simulink model "arcelik_a_senem_model"  (R2018b)
settings: Solver=FixedStepAuto  StartTime=0.0  StopTime=10  FixedStep=Tss  MaxStep=5e-5  RelTol=1e-3
undefined symbols (not defined in the file): Fs, polePairs, Tmax, Ts, Tss, Vdc, Wmax
libraries: simulink x1
settings Model: Creator=26046633  LastModifiedBy=26046633
settings SolverCC: ZeroCrossAlgorithm=Adaptive  AutoInsertRateTranBlk=on
settings DataIOCC: ReturnWorkspaceOutputs=on
settings DebuggingCC: IgnoredZcDiagnostic=none

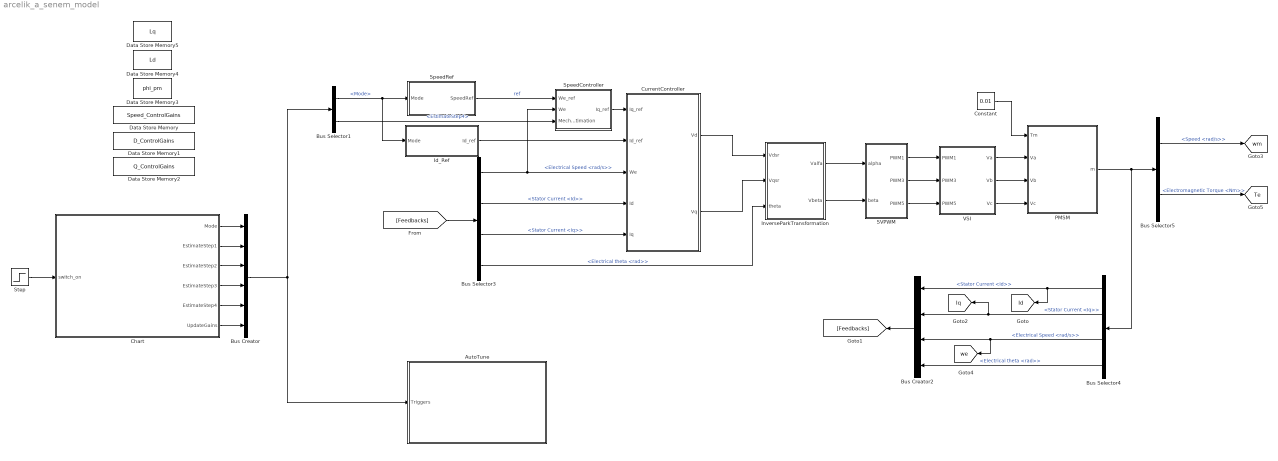
== system arcelik_a_senem_model ==
  AutoTune : Subsystem
  Bus Creator : BusCreator  Inputs=6
  Bus Creator2 : BusCreator  Inputs=4
  Bus Selector1 : BusSelector  OutputSignals=Mode,EstimateStep4
  Bus Selector3 : BusSelector  OutputSignals=Electrical Speed <rad/s>,Stator Current <Id>,Stator Current <Iq>,Electrical theta <rad>
  Bus Selector4 : BusSelector  OutputSignals=Stator Current <Id>,Stator Current <Iq>,Electrical Speed <rad/s>,Electrical theta <rad>
  Bus Selector5 : BusSelector  OutputSignals=Speed <rad/s>,Electromagnetic Torque <Nm>
  Chart : Stateflow chart  TreatAsAtomicUnit=on
  Constant : Constant  Value=0.01
  CurrentController : Subsystem
  Data Store Memory : DataStoreMemory  DataStoreName=Speed_ControlGains  InitialValue=[1 0]  ShowAdditionalParam=off
  Data Store Memory1 : DataStoreMemory  DataStoreName=D_ControlGains  InitialValue=[1 0]  ShowAdditionalParam=off
  Data Store Memory2 : DataStoreMemory  DataStoreName=Q_ControlGains  InitialValue=[1 0]  ShowAdditionalParam=off
  Data Store Memory3 : DataStoreMemory  DataStoreName=phi_pm  InitialValue=0.1  ShowAdditionalParam=off
  Data Store Memory4 : DataStoreMemory  DataStoreName=Ld  InitialValue=0.001  ShowAdditionalParam=off
  Data Store Memory5 : DataStoreMemory  DataStoreName=Lq  InitialValue=0.001  ShowAdditionalParam=off
  Id_Ref : Subsystem
  InverseParkTransformation : Subsystem
  PMSM : Subsystem  mask(Permanent Magnet Synchronous Motor :){Rs=7.1, Ld=30e-3, Lq=30e-3, flux=0.2, J=5.8e-4, B=2e-3, p=3}
      mask prompts: Rs "Stator Resistance - Rs [ohm] :"; Ld "Direct axis Inductance - Ld [H]"; Lq "Quadrature axis Inductance - Lq [H] :"; flux "Flux - [Wb]"; J "Rotor Inertia - J [kg-m^2]"; B "Friction Coefficient - B"; p "Number of Pole Pairs"
      mask Display: fprintf('PMSM')
  SVPWM : Subsystem
  SpeedController : Subsystem
  SpeedRef : Subsystem
  Step : Step  Time=3  Before=1  After=0  SampleTime=0
  VSI : Subsystem
  tag scope: Id=global, Iq=global, Te=global, we=global, wm=global
  wires:
  SVPWM/3(PWM5) -> VSI/3(PWM5)
  SVPWM/1(PWM1) -> VSI/1(PWM1)
  SVPWM/2(PWM3) -> VSI/2(PWM3)
  VSI/1(Va) -> PMSM/2(Va)
  VSI/2(Vb) -> PMSM/3(Vb)
  VSI/3(Vc) -> PMSM/4(Vc)
  SpeedController/1(Iq_ref) -> CurrentController/1(Iq_ref)
  SpeedRef/1(SpeedRef) -> SpeedController/1(We_ref)  "ref"
  Step/1 -> Chart/1(switch_on)
  Id_Ref/1(Id_ref) -> CurrentController/2(Id_ref)
  Chart/1(Mode) -> Bus Creator/1
  Chart/2(EstimateStep1) -> Bus Creator/2
  Chart/3(EstimateStep2) -> Bus Creator/3
  Chart/4(EstimateStep3) -> Bus Creator/4
  Bus Creator/1 -> AutoTune/1(Triggers), Bus Selector1/1
  Bus Selector1/1 -> Id_Ref/1(Mode), SpeedRef/1(Mode)  "<Mode>"
  [Feedbacks] -> Bus Selector3/1
  Bus Selector3/4 -> InverseParkTransformation/3(theta)  "<Electrical theta <rad>>"
  Bus Selector3/1 -> SpeedController/2(We), CurrentController/3(We)  "<Electrical Speed <rad/s>>"
  Bus Selector3/2 -> CurrentController/4(Id)  "<Stator Current <Id>>"
  Bus Selector3/3 -> CurrentController/5(Iq)  "<Stator Current <Iq>>"
  PMSM/1(m) -> Bus Selector4/1, Bus Selector5/1
  InverseParkTransformation/1(Valfa) -> SVPWM/1(alpha)
  InverseParkTransformation/2(Vbeta) -> SVPWM/2(beta)
  CurrentController/2(Vq) -> InverseParkTransformation/2(Vqsr)
  CurrentController/1(Vd) -> InverseParkTransformation/1(Vdsr)
  Bus Creator2/1 -> [Feedbacks]
  Constant/1 -> PMSM/1(Tm)
  Bus Selector4/1 -> Bus Creator2/1, [Id]  "<Stator Current <Id>>"
  Bus Selector4/4 -> Bus Creator2/4  "<Electrical theta <rad>>"
  Bus Selector4/3 -> Bus Creator2/3, [we]  "<Electrical Speed <rad/s>>"
  Bus Selector4/2 -> [Iq], Bus Creator2/2  "<Stator Current <Iq>>"
  Bus Selector5/2 -> [Te]  "<Electromagnetic Torque <Nm>>"
  Bus Selector1/2 -> SpeedController/3(MechanicalEstimation)  "<EstimateStep4>"
  Bus Selector5/1 -> [wm]  "<Speed <rad/s>>"
  Chart/5(EstimateStep4) -> Bus Creator/5
  Chart/6(UpdateGains) -> Bus Creator/6

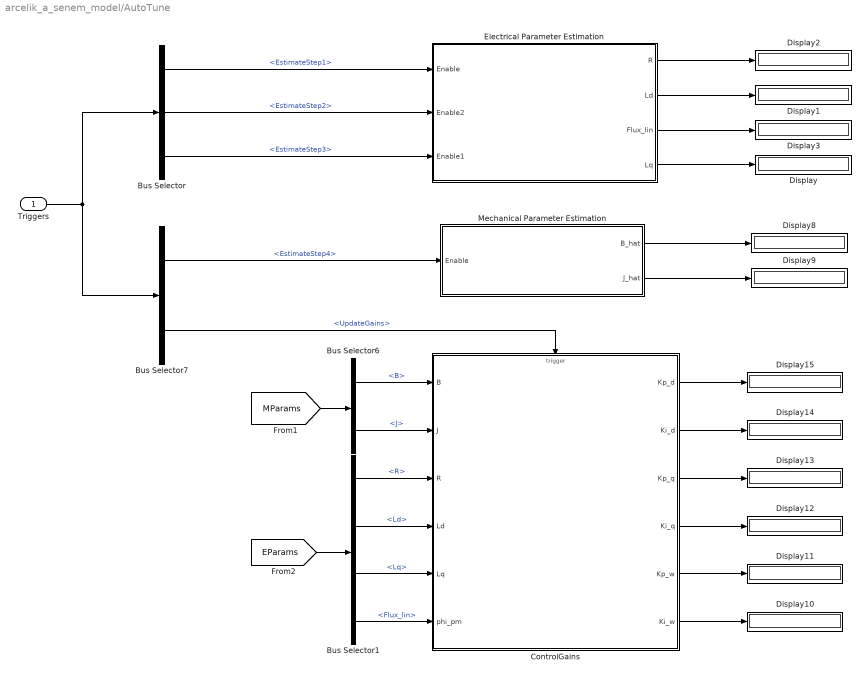
== system arcelik_a_senem_model/AutoTune ==
  Triggers : Inport
  Bus Selector : BusSelector  OutputSignals=EstimateStep1,EstimateStep2,EstimateStep3
  Bus Selector1 : BusSelector  OutputSignals=R,Ld,Lq,Flux_lin
  Bus Selector6 : BusSelector  OutputSignals=B,J
  Bus Selector7 : BusSelector  OutputSignals=EstimateStep4,UpdateGains
  ControlGains : Subsystem
  Display{,1..3,8..15} (12 alike) : Display
      Display1 settings: Decimation=4
  Electrical Parameter Estimation : Subsystem
  Mechanical Parameter Estimation : Subsystem
  wires:
  ControlGains/5(Kp_w) -> Display11/1
  Bus Selector/2 -> Electrical Parameter Estimation/2(Enable2)  "<EstimateStep2>"
  Electrical Parameter Estimation/2(Ld) -> Display1/1
  Mechanical Parameter Estimation/2(J_hat) -> Display9/1
  Electrical Parameter Estimation/1(R) -> Display2/1
  Bus Selector7/1 -> Mechanical Parameter Estimation/1(Enable)  "<EstimateStep4>"
  Bus Selector/3 -> Electrical Parameter Estimation/3(Enable1)  "<EstimateStep3>"
  Bus Selector/1 -> Electrical Parameter Estimation/1(Enable)  "<EstimateStep1>"
  Electrical Parameter Estimation/3(Flux_lin) -> Display3/1
  Electrical Parameter Estimation/4(Lq) -> Display/1
  Triggers/1 -> Bus Selector/1, Bus Selector7/1
  ControlGains/6(Ki_w) -> Display10/1
  [MParams] -> Bus Selector6/1
  Mechanical Parameter Estimation/1(B_hat) -> Display8/1
  Bus Selector7/2 -> ControlGains/Trigger  "<UpdateGains>"
  Bus Selector1/3 -> ControlGains/5(Lq)  "<Lq>"
  Bus Selector1/2 -> ControlGains/4(Ld)  "<Ld>"
  [EParams] -> Bus Selector1/1
  Bus Selector1/1 -> ControlGains/3(R)  "<R>"
  ControlGains/4(Ki_q) -> Display12/1
  ControlGains/3(Kp_q) -> Display13/1
  ControlGains/2(Ki_d) -> Display14/1
  ControlGains/1(Kp_d) -> Display15/1
  Bus Selector6/1 -> ControlGains/1(B)  "<B>"
  Bus Selector6/2 -> ControlGains/2(J)  "<J>"
  Bus Selector1/4 -> ControlGains/6(phi_pm)  "<Flux_lin>"

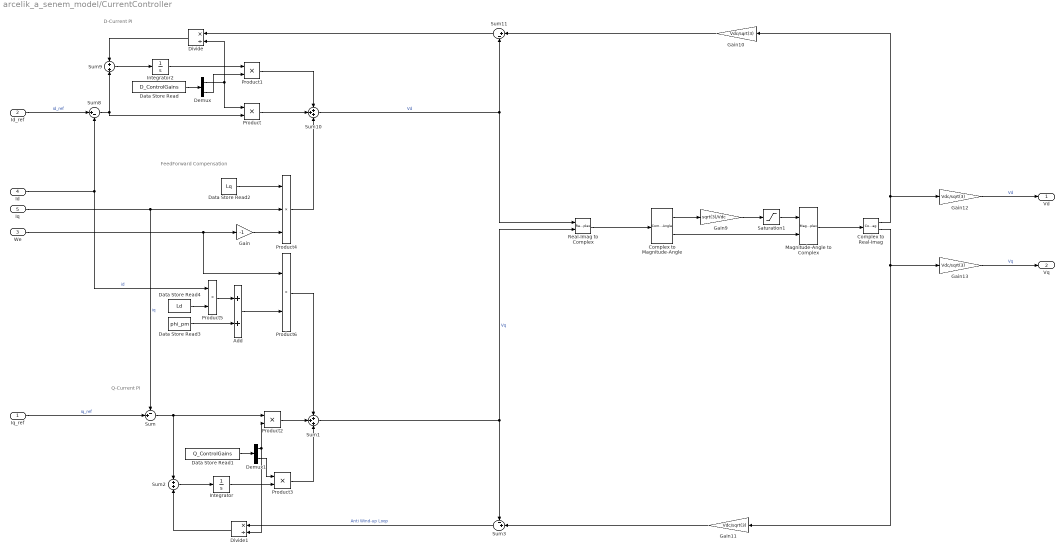
== system arcelik_a_senem_model/CurrentController ==
  note: FeedForward Compensation
  note: Q-Current PI
  note: D-Current PI
  Iq_ref : Inport
  Id_ref : Inport  Port=2
  We : Inport  Port=3
  Id : Inport  Port=4
  Iq : Inport  Port=5
  Add : Sum
  Complex to Magnitude-Angle : ComplexToMagnitudeAngle
  Complex to Real-Imag : ComplexToRealImag
  Data Store Read : DataStoreRead  DataStoreName=D_ControlGains
  Data Store Read1 : DataStoreRead  DataStoreName=Q_ControlGains
  Data Store Read2 : DataStoreRead  DataStoreName=Lq
  Data Store Read3 : DataStoreRead  DataStoreName=phi_pm
  Data Store Read4 : DataStoreRead  DataStoreName=Ld
  Demux : Demux  Outputs=2
  Demux1 : Demux  Outputs=2
  Divide : Product  Inputs=*/
  Divide1 : Product  Inputs=*/
  Gain : Gain  Gain=-1
  Gain{10..13} (4 alike) : Gain  Gain=Vdc/sqrt(3)
  Gain9 : Gain  Gain=sqrt(3)/Vdc
  Integrator : Integrator
  Integrator2 : Integrator
  Magnitude-Angle to Complex : MagnitudeAngleToComplex
  Product{,1..3,5..6} (6 alike) : Product
  Product4 : Product  Inputs=3
  Real-Imag to Complex : RealImagToComplex
  Saturation1 : Saturate  UpperLimit=sqrt(3)*2/3  LowerLimit=-sqrt(3)*2/3
  Sum : Sum  Inputs=-+|
  Sum1 : Sum  Inputs=+++
  Sum10 : Sum  Inputs=+++
  Sum11 : Sum  Inputs=|+-
  Sum2 : Sum
  Sum3 : Sum  Inputs=-+|
  Sum8 : Sum  Inputs=|+-
  Sum9 : Sum  Inputs=+|+
  Vd : Outport
  Vq : Outport  Port=2
  wires:
  Integrator2/1 -> Product1/1
  Sum/1 -> Sum2/1, Product2/1
  Product6/1 -> Sum1/1
  Integrator/1 -> Product3/2
  Sum2/1 -> Integrator/1
  Sum8/1 -> Product/2, Sum9/2
  Product4/1 -> Sum10/3
  Product3/1 -> Sum1/3
  Id/1 -> Sum8/2, Product5/1  "id"
  Divide/1 -> Sum9/1
  Iq/1 -> Sum/1, Product4/2  "iq"
  Product1/1 -> Sum10/1
  Product2/1 -> Sum1/2
  Divide1/1 -> Sum2/2
  Id_ref/1 -> Sum8/1  "id_ref"
  Sum9/1 -> Integrator2/1
  Product/1 -> Sum10/2
  We/1 -> Product6/1, Gain/1
  Complex to Magnitude-Angle/2 -> Magnitude-Angle to Complex/2
  Sum11/1 -> Divide/1
  Gain11/1 -> Sum3/2
  Real-Imag to Complex/1 -> Complex to Magnitude-Angle/1
  Gain10/1 -> Sum11/1
  Gain9/1 -> Saturation1/1
  Complex to Magnitude-Angle/1 -> Gain9/1
  Gain13/1 -> Vq/1  "Vq"
  Sum3/1 -> Divide1/1  "Anti Wind-up Loop"
  Complex to Real-Imag/2 -> Gain13/1, Gain11/1
  Sum1/1 -> Sum3/1, Real-Imag to Complex/2  "Vq"
  Complex to Real-Imag/1 -> Gain10/1, Gain12/1
  Magnitude-Angle to Complex/1 -> Complex to Real-Imag/1
  Sum10/1 -> Real-Imag to Complex/1, Sum11/2  "Vd"
  Saturation1/1 -> Magnitude-Angle to Complex/1
  Iq_ref/1 -> Sum/2  "iq_ref"
  Gain12/1 -> Vd/1  "Vd"
  Data Store Read/1 -> Demux/1
  Demux/1 -> Divide/2, Product/1
  Demux/2 -> Product1/2
  Data Store Read1/1 -> Demux1/1
  Demux1/1 -> Product2/2, Divide1/2
  Demux1/2 -> Product3/1
  Data Store Read2/1 -> Product4/1
  Gain/1 -> Product4/3
  Data Store Read4/1 -> Product5/2
  Product5/1 -> Add/1
  Data Store Read3/1 -> Add/2
  Add/1 -> Product6/2

== system arcelik_a_senem_model/Id_Ref ==
  Mode : Inport
  Constant1 : Constant  Value=0
  Multiport Switch1 : MultiPortSwitch  Inputs=4
  Sine Wave : Sin  Amplitude=0.1  Frequency=100*2*pi  SampleTime=0
  Sine Wave1 : Sin  Amplitude=0.1  Frequency=500*2*pi  SampleTime=0
  Sum : Sum
  Id_ref : Outport
  wires:
  Multiport Switch1/1 -> Id_ref/1
  Sum/1 -> Multiport Switch1/2
  Sine Wave/1 -> Sum/1
  Sine Wave1/1 -> Sum/2
  Mode/1 -> Multiport Switch1/1
  Constant1/1 -> Multiport Switch1/5, Multiport Switch1/4, Multiport Switch1/3

== system arcelik_a_senem_model/InverseParkTransformation ==
  Vdsr : Inport
  Vqsr : Inport  Port=2
  theta : Inport  Port=3
  ipark : MATLAB Function  TreatAsAtomicUnit=on  SystemSampleTime=Ts
  Valfa : Outport  VectorParamsAs1DForOutWhenUnconnected=off
  Vbeta : Outport  Port=2  VectorParamsAs1DForOutWhenUnconnected=off
  wires:
  theta/1 -> ipark/3(Angle)
  ipark/1(Alpha) -> Valfa/1
  ipark/2(Beta) -> Vbeta/1
  Vdsr/1 -> ipark/1(Ds)
  Vqsr/1 -> ipark/2(Qs)

== system arcelik_a_senem_model/PMSM ==
  Tm : Inport
  Va : Inport  Port=2
  Vb : Inport  Port=3
  Vc : Inport  Port=4
  Clark & Park Tranformations : Subsystem
  "Id, Iq Calculation" : Subsystem
  Mechanical Calculation : Subsystem
  Torque Calculation : Subsystem
  measurement : Subsystem
  m : Outport
  tag scope: Vd=global, Vq=global
  wires:
  Tm/1 -> Mechanical Calculation/2(Tm)
  Torque Calculation/1(Te) -> measurement/3(Te), Mechanical Calculation/1(Te)
  Mechanical Calculation/4(we) -> "Id, Iq Calculation"/3(we), measurement/7(we)
  Mechanical Calculation/3(theta) -> Clark & Park Tranformations/4(theta), measurement/6(theta_e)
  "Id, Iq Calculation"/1(Iq) -> measurement/2(Iq), Torque Calculation/1(Iq)
  Mechanical Calculation/1(wm) -> measurement/4(wm)
  Mechanical Calculation/2(theta m) -> measurement/5(theta_m)
  measurement/1(m) -> m/1
  Clark & Park Tranformations/1(Vq) -> [Vq], "Id, Iq Calculation"/1(Vq)
  Clark & Park Tranformations/2(Vd) -> [Vd], "Id, Iq Calculation"/2(Vd)
  Va/1 -> Clark & Park Tranformations/1(Va)
  Vc/1 -> Clark & Park Tranformations/3(Vc)
  Vb/1 -> Clark & Park Tranformations/2(Vb)
  "Id, Iq Calculation"/2(Id) -> measurement/1(Id), Torque Calculation/2(Id)

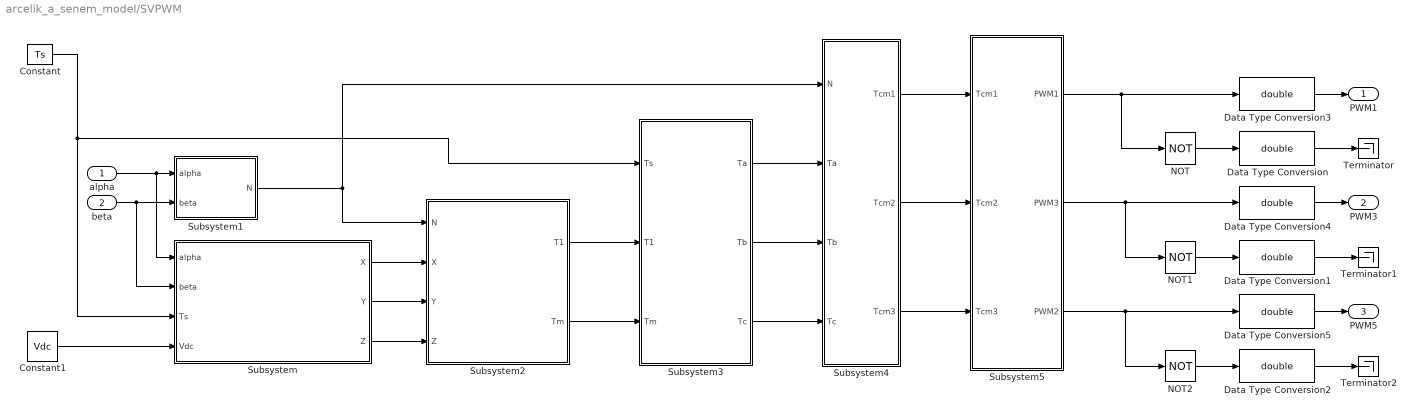
== system arcelik_a_senem_model/SVPWM ==
  alpha : Inport
  beta : Inport  Port=2
  Constant : Constant  Value=Ts
  Constant1 : Constant  Value=Vdc
  Data Type Conversion{,1..5} (6 alike) : DataTypeConversion  OutDataTypeStr=double
  NOT : Logic  Operator=NOT  AllPortsSameDT=off  OutDataTypeStr=boolean
  NOT1 : Logic  Operator=NOT  AllPortsSameDT=off  OutDataTypeStr=boolean
  NOT2 : Logic  Operator=NOT  AllPortsSameDT=off  OutDataTypeStr=boolean
  Subsystem : Subsystem
  Subsystem1 : Subsystem
  Subsystem2 : Subsystem
  Subsystem3 : Subsystem
  Subsystem4 : Subsystem
  Subsystem5 : Subsystem
  Terminator : Terminator
  Terminator1 : Terminator
  Terminator2 : Terminator
  PWM1 : Outport
  PWM3 : Outport  Port=2
  PWM5 : Outport  Port=3
  wires:
  Subsystem5/3(PWM2) -> Data Type Conversion5/1, NOT2/1
  NOT2/1 -> Data Type Conversion2/1
  NOT1/1 -> Data Type Conversion1/1
  NOT/1 -> Data Type Conversion/1
  Subsystem3/3(Tc) -> Subsystem4/4(Tc)
  Subsystem3/1(Ta) -> Subsystem4/2(Ta)
  Subsystem5/2(PWM3) -> Data Type Conversion4/1, NOT1/1
  Subsystem5/1(PWM1) -> Data Type Conversion3/1, NOT/1
  Subsystem4/3(Tcm3) -> Subsystem5/3(Tcm3)
  Subsystem4/2(Tcm2) -> Subsystem5/2(Tcm2)
  Subsystem4/1(Tcm1) -> Subsystem5/1(Tcm1)
  Subsystem3/2(Tb) -> Subsystem4/3(Tb)
  Constant/1 -> Subsystem3/1(Ts), Subsystem/3(Ts)
  Constant1/1 -> Subsystem/4(Vdc)
  beta/1 -> Subsystem1/2(beta), Subsystem/2(beta)
  Subsystem1/1(N) -> Subsystem4/1(N), Subsystem2/1(N)
  alpha/1 -> Subsystem1/1(alpha), Subsystem/1(alpha)
  Subsystem/2(Y) -> Subsystem2/3(Y)
  Subsystem/1(X) -> Subsystem2/2(X)
  Subsystem2/2(Tm) -> Subsystem3/3(Tm)
  Subsystem2/1(T1) -> Subsystem3/2(T1)
  Subsystem/3(Z) -> Subsystem2/4(Z)
  Data Type Conversion3/1 -> PWM1/1
  Data Type Conversion4/1 -> PWM3/1
  Data Type Conversion5/1 -> PWM5/1
  Data Type Conversion/1 -> Terminator/1
  Data Type Conversion1/1 -> Terminator1/1
  Data Type Conversion2/1 -> Terminator2/1

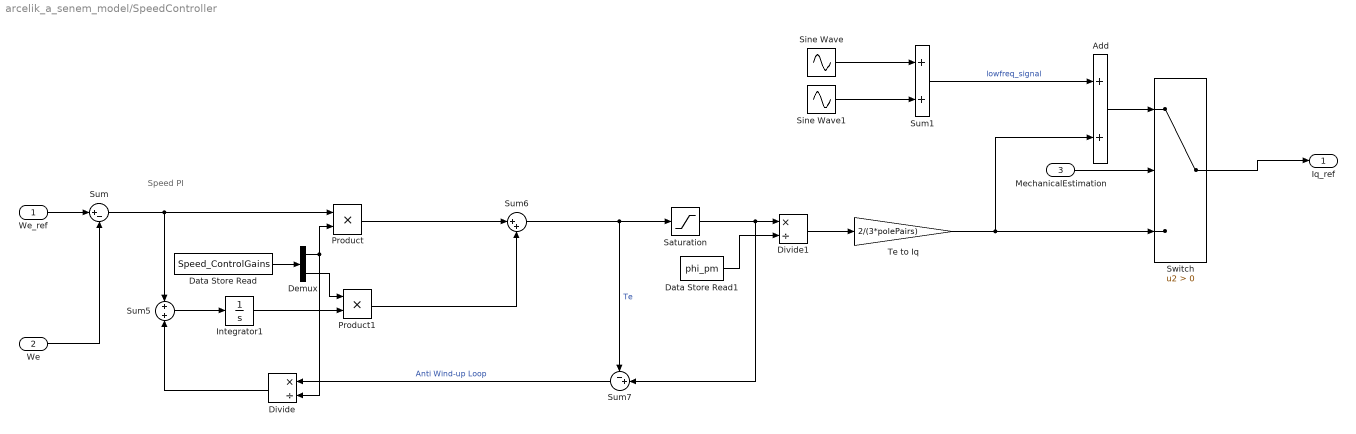
== system arcelik_a_senem_model/SpeedController ==
  note: Speed PI
  We_ref : Inport
  We : Inport  Port=2
  MechanicalEstimation : Inport  Port=3
  Add : Sum
  Data Store Read : DataStoreRead  DataStoreName=Speed_ControlGains
  Data Store Read1 : DataStoreRead  DataStoreName=phi_pm
  Demux : Demux  Outputs=2
  Divide : Product  Inputs=*/
  Divide1 : Product  Inputs=*/
  Integrator1 : Integrator
  Product : Product
  Product1 : Product
  Saturation : Saturate  UpperLimit=Tmax  LowerLimit=-Tmax
  Sine Wave : Sin  Amplitude=0.1  Frequency=0.1*2*pi  SampleTime=0
  Sine Wave1 : Sin  Amplitude=0.1  Frequency=0.25*2*pi  SampleTime=0
  Sum : Sum  Inputs=|+-
  Sum1 : Sum
  Sum5 : Sum
  Sum6 : Sum  Inputs=|++
  Sum7 : Sum  Inputs=-+|
  Switch : Switch  Criteria=u2 > Threshold
  Te to Iq : Gain  Gain=2/(3*polePairs)
  Iq_ref : Outport
  wires:
  Product1/1 -> Sum6/2
  Sum5/1 -> Integrator1/1
  Saturation/1 -> Sum7/2, Divide1/1
  Integrator1/1 -> Product1/2
  Sum6/1 -> Saturation/1, Sum7/1  "Te"
  Sum7/1 -> Divide/1  "Anti Wind-up Loop"
  Product/1 -> Sum6/1
  Divide/1 -> Sum5/2
  Sum/1 -> Sum5/1, Product/1
  We_ref/1 -> Sum/1
  We/1 -> Sum/2
  Te to Iq/1 -> Add/2, Switch/3
  Switch/1 -> Iq_ref/1
  Sine Wave1/1 -> Sum1/2
  Sine Wave/1 -> Sum1/1
  MechanicalEstimation/1 -> Switch/2
  Add/1 -> Switch/1
  Sum1/1 -> Add/1  "lowfreq_signal"
  Data Store Read/1 -> Demux/1
  Demux/2 -> Product1/1
  Demux/1 -> Product/2, Divide/2
  Divide1/1 -> Te to Iq/1
  Data Store Read1/1 -> Divide1/2

== system arcelik_a_senem_model/SpeedRef ==
  Mode : Inport
  Constant : Constant  Value=100
  Constant1 : Constant  Value=2500
  Constant2 : Constant  Value=Wmax
  Constant3 : Constant  Value=0
  Gain : Gain  Gain=Wmax
  Gain1 : Gain  Gain=pi/(30*Wmax)
  Gain2 : Gain  Gain=pi/(30*Wmax)
  Gain3 : Gain  Gain=pi/(30*Wmax)
  Multiport Switch : MultiPortSwitch  Inputs=4
  RC_MACRO1 : MATLAB Function  TreatAsAtomicUnit=on  SystemSampleTime=Ts
  Step : Step  Time=5.5  After=1000  SampleTime=0
  SpeedRef : Outport
  wires:
  Constant/1 -> Gain1/1  "rpm"
  Mode/1 -> Multiport Switch/1
  Constant3/1 -> Multiport Switch/2
  Step/1 -> Gain3/1
  Constant1/1 -> Gain2/1  "rpm"
  RC_MACRO1/1(SetpointValue) -> Gain/1
  Multiport Switch/1 -> RC_MACRO1/1(inp)  "rad/s"
  Constant2/1 -> RC_MACRO1/2(MaxSpeed)
  Gain/1 -> SpeedRef/1
  Gain1/1 -> Multiport Switch/3  "rad/s"
  Gain2/1 -> Multiport Switch/4  "rad/s"
  Gain3/1 -> Multiport Switch/5  "rad/s"

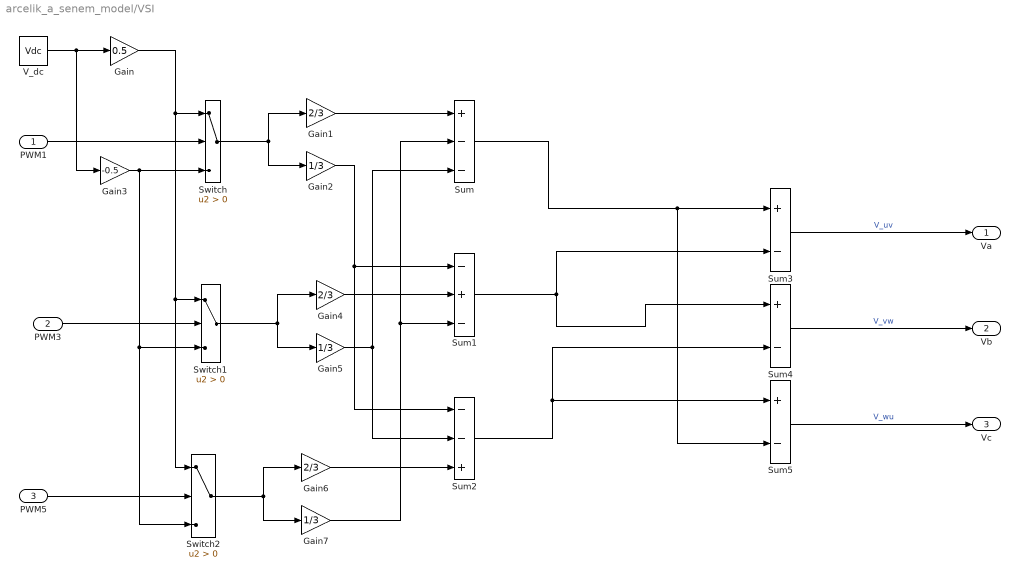
== system arcelik_a_senem_model/VSI ==
  PWM1 : Inport
  PWM3 : Inport  Port=2
  PWM5 : Inport  Port=3
  Gain : Gain  Gain=0.5
  Gain1 : Gain  Gain=2/3
  Gain2 : Gain  Gain=1/3
  Gain3 : Gain  Gain=-0.5
  Gain4 : Gain  Gain=2/3
  Gain5 : Gain  Gain=1/3
  Gain6 : Gain  Gain=2/3
  Gain7 : Gain  Gain=1/3
  Sum : Sum  Inputs=+--
  Sum1 : Sum  Inputs=-+-
  Sum2 : Sum  Inputs=--+
  Sum3 : Sum  Inputs=+-
  Sum4 : Sum  Inputs=+-
  Sum5 : Sum  Inputs=+-
  Switch : Switch  Criteria=u2 > Threshold
  Switch1 : Switch  Criteria=u2 > Threshold
  Switch2 : Switch  Criteria=u2 > Threshold
  V_dc : Constant  Value=Vdc
  Va : Outport
  Vb : Outport  Port=2
  Vc : Outport  Port=3
  wires:
  V_dc/1 -> Gain3/1, Gain/1
  PWM1/1 -> Switch/2
  Switch/1 -> Gain2/1, Gain1/1
  Gain1/1 -> Sum/1
  Sum/1 -> Sum5/2, Sum3/1
  PWM3/1 -> Switch1/2
  Sum1/1 -> Sum3/2, Sum4/1
  Switch1/1 -> Gain4/1, Gain5/1
  Gain4/1 -> Sum1/2
  Switch2/1 -> Gain7/1, Gain6/1
  Sum2/1 -> Sum4/2, Sum5/1
  Gain3/1 -> Switch2/3, Switch1/3, Switch/3
  PWM5/1 -> Switch2/2
  Gain/1 -> Switch2/1, Switch1/1, Switch/1
  Gain6/1 -> Sum2/3
  Gain7/1 -> Sum1/3, Sum/2
  Gain5/1 -> Sum/3, Sum2/2
  Gain2/1 -> Sum2/1, Sum1/1
  Sum3/1 -> Va/1  "V_uv"
  Sum4/1 -> Vb/1  "V_vw"
  Sum5/1 -> Vc/1  "V_wu"

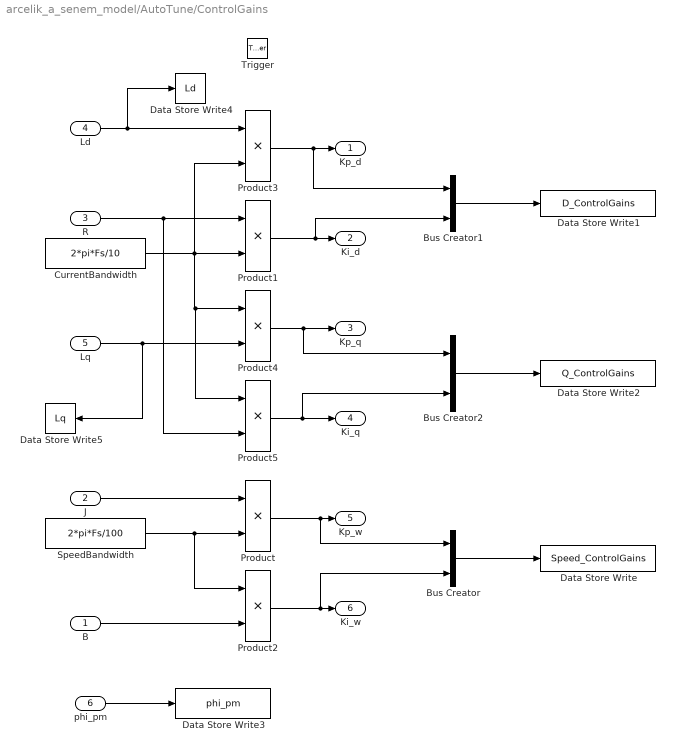
== system arcelik_a_senem_model/AutoTune/ControlGains ==
  B : Inport
  J : Inport  Port=2
  R : Inport  Port=3
  Ld : Inport  Port=4
  Lq : Inport  Port=5
  phi_pm : Inport  Port=6
  Trigger : TriggerPort  VariantControl=Variant  PortDimensions=1
  Bus Creator : BusCreator  Inputs=2
  Bus Creator1 : BusCreator  Inputs=2
  Bus Creator2 : BusCreator  Inputs=2
  CurrentBandwidth : Constant  Value=2*pi*Fs/10
  Data Store Write : DataStoreWrite  DataStoreName=Speed_ControlGains
  Data Store Write1 : DataStoreWrite  DataStoreName=D_ControlGains
  Data Store Write2 : DataStoreWrite  DataStoreName=Q_ControlGains
  Data Store Write3 : DataStoreWrite  DataStoreName=phi_pm
  Data Store Write4 : DataStoreWrite  DataStoreName=Ld
  Data Store Write5 : DataStoreWrite  DataStoreName=Lq
  Product{,1..5} (6 alike) : Product
  SpeedBandwidth : Constant  Value=2*pi*Fs/100
  Kp_d : Outport
  Ki_d : Outport  Port=2
  Kp_q : Outport  Port=3
  Ki_q : Outport  Port=4
  Kp_w : Outport  Port=5
  Ki_w : Outport  Port=6
  wires:
  B/1 -> Product2/2
  SpeedBandwidth/1 -> Product/2, Product2/1
  J/1 -> Product/1
  Bus Creator/1 -> Data Store Write/1
  Product2/1 -> Bus Creator/2, Ki_w/1
  Bus Creator1/1 -> Data Store Write1/1
  Bus Creator2/1 -> Data Store Write2/1
  Lq/1 -> Data Store Write5/1, Product4/2
  Product5/1 -> Bus Creator2/2, Ki_q/1
  Ld/1 -> Data Store Write4/1, Product3/1
  CurrentBandwidth/1 -> Product5/1, Product4/1, Product3/2, Product1/2
  Product1/1 -> Bus Creator1/2, Ki_d/1
  R/1 -> Product5/2, Product1/1
  Product3/1 -> Bus Creator1/1, Kp_d/1
  Product4/1 -> Bus Creator2/1, Kp_q/1
  Product/1 -> Bus Creator/1, Kp_w/1
  phi_pm/1 -> Data Store Write3/1

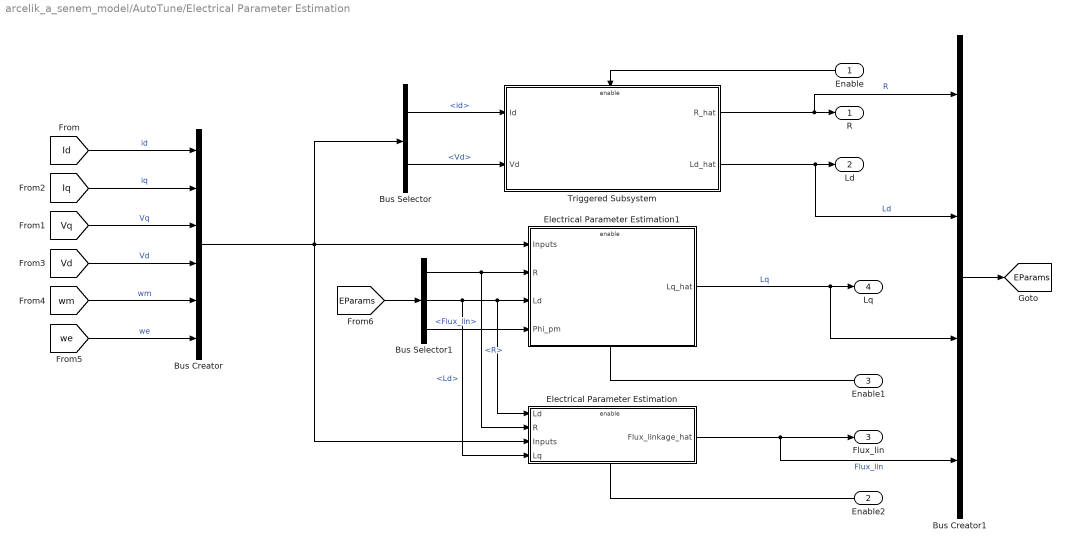
== system arcelik_a_senem_model/AutoTune/Electrical Parameter Estimation ==
  Enable : Inport
  Enable2 : Inport  Port=2
  Enable1 : Inport  Port=3
  Bus Creator : BusCreator  Inputs=6
  Bus Creator1 : BusCreator  Inputs=4
  Bus Selector : BusSelector  OutputSignals=id,Vd
  Bus Selector1 : BusSelector  OutputSignals=R,Ld,Flux_lin
  Electrical Parameter Estimation : Subsystem
  Electrical Parameter Estimation1 : Subsystem
  Triggered Subsystem : Subsystem  TreatAsAtomicUnit=on
  R : Outport
  Ld : Outport  Port=2
  Flux_lin : Outport  Port=3
  Lq : Outport  Port=4
  tag scope: EParams=global
  wires:
  [Vq] -> Bus Creator/3  "Vq"
  Bus Creator/1 -> Electrical Parameter Estimation/3(Inputs), Electrical Parameter Estimation1/1(Inputs), Bus Selector/1
  [we] -> Bus Creator/6  "we"
  [Id] -> Bus Creator/1  "id"
  [wm] -> Bus Creator/5  "wm"
  Bus Selector/1 -> Triggered Subsystem/1(Id)  "<id>"
  [Iq] -> Bus Creator/2  "iq"
  Bus Selector/2 -> Triggered Subsystem/2(Vd)  "<Vd>"
  Enable1/1 -> Electrical Parameter Estimation1/Enable
  [Vd] -> Bus Creator/4  "Vd"
  Electrical Parameter Estimation/1(Flux_linkage_hat) -> Flux_lin/1, Bus Creator1/4  "Flux_lin"
  Enable2/1 -> Electrical Parameter Estimation/Enable
  Electrical Parameter Estimation1/1(Lq_hat) -> Bus Creator1/3, Lq/1  "Lq"
  Triggered Subsystem/1(R_hat) -> Bus Creator1/1, R/1  "R"
  Triggered Subsystem/2(Ld_hat) -> Bus Creator1/2, Ld/1  "Ld"
  Bus Creator1/1 -> [EParams]
  [EParams] -> Bus Selector1/1
  Bus Selector1/1 -> Electrical Parameter Estimation/2(R), Electrical Parameter Estimation1/2(R)  "<R>"
  Bus Selector1/2 -> Electrical Parameter Estimation/4(Lq), Electrical Parameter Estimation/1(Ld), Electrical Parameter Estimation1/3(Ld)  "<Ld>"
  Bus Selector1/3 -> Electrical Parameter Estimation1/4(Phi_pm)  "<Flux_lin>"
  Enable/1 -> Triggered Subsystem/Enable

== system arcelik_a_senem_model/AutoTune/Mechanical Parameter Estimation ==
  Enable : Inport
  Bus Creator : BusCreator  Inputs=2
  Mechanical Parameter Estimation : Subsystem
  B_hat : Outport
  J_hat : Outport  Port=2
  tag scope: MParams=global
  wires:
  [wm] -> Mechanical Parameter Estimation/1(wm)
  Mechanical Parameter Estimation/2(J_hat) -> Bus Creator/2, J_hat/1  "J"
  Mechanical Parameter Estimation/1(B_hat) -> Bus Creator/1, B_hat/1  "B"
  Enable/1 -> Mechanical Parameter Estimation/Enable
  [Te] -> Mechanical Parameter Estimation/2(Te)
  Bus Creator/1 -> [MParams]

== system arcelik_a_senem_model/PMSM/Clark & Park Tranformations ==
  Va : Inport
  Vb : Inport  Port=2
  Vc : Inport  Port=3
  theta : Inport  Port=4
  Fcn : Fcn  Expr=u(1)*cos(u(4))+u(2)*cos(u(4)-2*pi/3)+u(3)*cos(u(4)+2*pi/3)
  Fcn1 : Fcn  Expr=-u(1)*sin(u(4))-u(2)*sin(u(4)-2*pi/3)-u(3)*sin(u(4)+2*pi/3)
  Gain : Gain  Gain=2/3
  Gain1 : Gain  Gain=2/3
  Mux : Mux  Inputs=2
  Mux1 : Mux  Inputs=2
  Mux3 : Mux  Inputs=3
  Vq : Outport
  Vd : Outport  Port=2
  wires:
  Mux3/1 -> Mux1/1, Mux/1
  Mux1/1 -> Fcn1/1
  theta/1 -> Mux1/2, Mux/2
  Mux/1 -> Fcn/1
  Va/1 -> Mux3/1
  Vb/1 -> Mux3/2
  Vc/1 -> Mux3/3
  Fcn/1 -> Gain/1
  Fcn1/1 -> Gain1/1
  Gain/1 -> Vd/1
  Gain1/1 -> Vq/1

== system arcelik_a_senem_model/PMSM/Id, Iq Calculation ==
  Vq : Inport
  Vd : Inport  Port=2
  we : Inport  Port=3
  Id cal : Subsystem
  Iq cal : Subsystem
  Iq : Outport
  Id : Outport  Port=2
  wires:
  Iq cal/1(Iq) -> Id cal/1(Iq), Iq/1
  Id cal/1(Id) -> Iq cal/1(Id), Id/1
  we/1 -> Iq cal/3(we), Id cal/2(we)
  Vq/1 -> Iq cal/2(Vq)
  Vd/1 -> Id cal/3(Vd)

== system arcelik_a_senem_model/PMSM/Mechanical Calculation ==
  Te : Inport
  Tm : Inport  Port=2
  1/J : Gain  Gain=1/J
  1/p : Gain  Gain=1/p
  B : Gain  Gain=B
  Integrator : Integrator
  Integrator1 : Integrator
  Sum : Sum  Inputs=-+-
  p : Gain  Gain=p
  wm : Outport
  theta m : Outport  Port=2
  theta : Outport  Port=3
  we : Outport  Port=4
  wires:
  Te/1 -> Sum/2
  Tm/1 -> Sum/1
  Sum/1 -> 1/J/1
  1/J/1 -> Integrator/1
  Integrator/1 -> B/1, p/1, wm/1
  B/1 -> Sum/3
  p/1 -> we/1, Integrator1/1
  Integrator1/1 -> theta/1, 1/p/1
  1/p/1 -> theta m/1

== system arcelik_a_senem_model/PMSM/Torque Calculation ==
  Iq : Inport
  Id : Inport  Port=2
  1.5 P : Gain  Gain=1.5*p
  Mux : Mux  Inputs=2
      settings: DisplayOption=signals
  Torque calculation : Fcn  Expr=flux*u(1)+(Ld - Lq)*u(1)*u*(2)
  Te : Outport
  wires:
  Torque calculation/1 -> Te/1  "Te"
  Mux/1 -> 1.5 P/1
  Iq/1 -> Mux/1  "Iq"
  Id/1 -> Mux/2  "Id"
  1.5 P/1 -> Torque calculation/1

== system arcelik_a_senem_model/PMSM/measurement ==
  Id : Inport
  Iq : Inport  Port=2
  Te : Inport  Port=3
  wm : Inport  Port=4
  theta_m : Inport  Port=5
  theta_e : Inport  Port=6
  we : Inport  Port=7
  Bus Creator : BusCreator  Inputs=7
  m : Outport
  wires:
  Id/1 -> Bus Creator/1  "Stator Current <Id>"
  Iq/1 -> Bus Creator/2  "Stator Current <Iq>"
  Te/1 -> Bus Creator/3  "Electromagnetic Torque <Nm>"
  wm/1 -> Bus Creator/4  "Speed <rad/s>"
  Bus Creator/1 -> m/1
  theta_m/1 -> Bus Creator/7  "Rotor theta <rad>"
  we/1 -> Bus Creator/5  "Electrical Speed <rad/s>"
  theta_e/1 -> Bus Creator/6  "Electrical theta <rad>"

== system arcelik_a_senem_model/SVPWM/Subsystem ==
  alpha : Inport
  beta : Inport  Port=2
  Ts : Inport  Port=3
  Vdc : Inport  Port=4
  Add : Sum
  Add1 : Sum  Inputs=-+
  Divide : Product  Inputs=**/
  Divide1 : Product  Inputs=**/
  Divide2 : Product  Inputs=**/
  Gain : Gain  Gain=2/sqrt(2)
  Gain1 : Gain  Gain=sqrt(3)
  Gain2 : Gain  Gain=1/sqrt(2)
  X : Outport
  Y : Outport  Port=2
  Z : Outport  Port=3
  wires:
  Add1/1 -> Divide2/1
  Divide2/1 -> Z/1
  Gain2/1 -> Divide1/2, Divide2/2
  Add/1 -> Divide1/1
  Divide1/1 -> Y/1
  Gain1/1 -> Add1/1, Add/1
  alpha/1 -> Gain1/1
  Gain/1 -> Divide/1
  Ts/1 -> Gain/1, Gain2/1
  beta/1 -> Divide/2, Add/2, Add1/2
  Vdc/1 -> Divide2/3, Divide1/3, Divide/3
  Divide/1 -> X/1

== system arcelik_a_senem_model/SVPWM/Subsystem1 ==
  alpha : Inport
  beta : Inport  Port=2
  Add : Sum  Inputs=+++
  Add1 : Sum
  Add2 : Sum  Inputs=+-
  Constant : Constant
  Constant1 : Constant  Value=0
  Gain : Gain  Gain=4
  Gain1 : Gain  Gain=sqrt(3)
  Gain2 : Gain  Gain=2
  Switch : Switch  Criteria=u2 > Threshold
  Switch1 : Switch  Criteria=u2 > Threshold
  Switch2 : Switch  Criteria=u2 > Threshold
  N : Outport
  wires:
  alpha/1 -> Gain1/1
  Switch2/1 -> Add/3
  Add/1 -> N/1
  Switch1/1 -> Gain/1
  Gain1/1 -> Add1/1, Add2/1
  Gain2/1 -> Add/1
  Switch/1 -> Gain2/1
  beta/1 -> Switch2/2, Add1/2, Add2/2
  Add2/1 -> Switch/2
  Constant/1 -> Switch1/3, Switch2/1, Switch/1
  Gain/1 -> Add/2
  Add1/1 -> Switch1/2
  Constant1/1 -> Switch1/1, Switch/3, Switch2/3

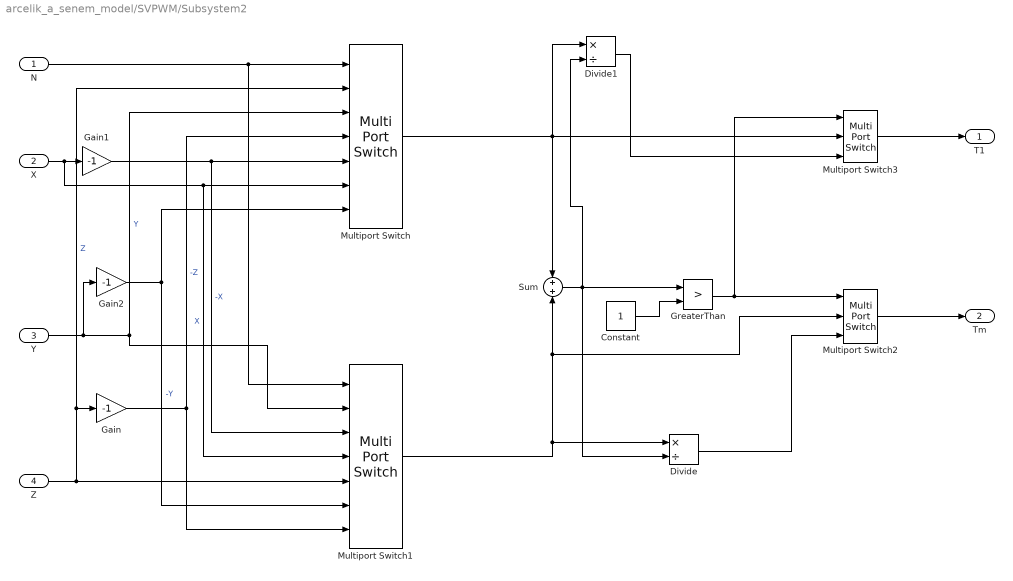
== system arcelik_a_senem_model/SVPWM/Subsystem2 ==
  N : Inport
  X : Inport  Port=2
  Y : Inport  Port=3
  Z : Inport  Port=4
  Constant : Constant
  Divide : Product  Inputs=*/
  Divide1 : Product  Inputs=*/
  Gain : Gain  Gain=-1
  Gain1 : Gain  Gain=-1
  Gain2 : Gain  Gain=-1
  GreaterThan : RelationalOperator  Operator=>  OutDataTypeStr=boolean  RndMeth=Simplest
  Multiport Switch : MultiPortSwitch  Inputs=6
  Multiport Switch1 : MultiPortSwitch  Inputs=6
  Multiport Switch2 : MultiPortSwitch  DataPortOrder=Zero-based contiguous  Inputs=2  zeroidx=on
  Multiport Switch3 : MultiPortSwitch  DataPortOrder=Zero-based contiguous  Inputs=2  zeroidx=on
  Sum : Sum  Inputs=+|+
  T1 : Outport
  Tm : Outport  Port=2
  wires:
  Multiport Switch2/1 -> Tm/1
  Multiport Switch3/1 -> T1/1
  GreaterThan/1 -> Multiport Switch2/1, Multiport Switch3/1
  Constant/1 -> GreaterThan/2
  Sum/1 -> GreaterThan/1, Divide/2, Divide1/2
  Multiport Switch1/1 -> Sum/2, Multiport Switch2/2, Divide/1
  Multiport Switch/1 -> Sum/1, Multiport Switch3/2, Divide1/1
  Gain2/1 -> Multiport Switch/7, Multiport Switch1/6  "-Y"
  Gain1/1 -> Multiport Switch/5, Multiport Switch1/3  "-X"
  X/1 -> Gain1/1, Multiport Switch/6, Multiport Switch1/4  "X"
  Gain/1 -> Multiport Switch/4, Multiport Switch1/7  "-Z"
  Y/1 -> Multiport Switch/3, Multiport Switch1/2, Gain2/1  "Y"
  Z/1 -> Multiport Switch1/5, Multiport Switch/2, Gain/1  "Z"
  N/1 -> Multiport Switch1/1, Multiport Switch/1
  Divide/1 -> Multiport Switch2/3
  Divide1/1 -> Multiport Switch3/3

== system arcelik_a_senem_model/SVPWM/Subsystem3 ==
  Ts : Inport
  T1 : Inport  Port=2
  Tm : Inport  Port=3
  Gain : Gain  Gain=0.25
  Gain1 : Gain  Gain=0.5
  Gain2 : Gain  Gain=0.5
  Sum : Sum  Inputs=+|+
  Sum1 : Sum  Inputs=+-|
  Sum2 : Sum  Inputs=|++
  Sum3 : Sum  Inputs=++|
  Ta : Outport
  Tb : Outport  Port=2
  Tc : Outport  Port=3
  wires:
  Gain2/1 -> Sum3/2
  Sum3/1 -> Tc/1
  Gain1/1 -> Sum2/1
  Sum2/1 -> Tb/1, Sum3/1
  Gain/1 -> Sum2/2, Ta/1
  Sum1/1 -> Gain/1
  Ts/1 -> Sum1/1
  Sum/1 -> Sum1/2
  Tm/1 -> Sum/2, Gain2/1
  T1/1 -> Gain1/1, Sum/1

== system arcelik_a_senem_model/SVPWM/Subsystem4 ==
  N : Inport
  Ta : Inport  Port=2
  Tb : Inport  Port=3
  Tc : Inport  Port=4
  Multiport Switch : MultiPortSwitch  Inputs=6
  Multiport Switch1 : MultiPortSwitch  Inputs=6
  Multiport Switch2 : MultiPortSwitch  Inputs=6
  Tcm1 : Outport
  Tcm2 : Outport  Port=2
  Tcm3 : Outport  Port=3
  wires:
  Multiport Switch2/1 -> Tcm3/1
  Multiport Switch1/1 -> Tcm2/1
  Tc/1 -> Multiport Switch2/2, Multiport Switch/5, Multiport Switch/6, Multiport Switch1/3, Multiport Switch1/7, Multiport Switch2/4
  Ta/1 -> Multiport Switch/3, Multiport Switch/4, Multiport Switch1/2, Multiport Switch1/6, Multiport Switch2/5, Multiport Switch2/7
  Tb/1 -> Multiport Switch2/3, Multiport Switch2/6, Multiport Switch1/4, Multiport Switch/2, Multiport Switch/7, Multiport Switch1/5
  N/1 -> Multiport Switch/1, Multiport Switch2/1, Multiport Switch1/1
  Multiport Switch/1 -> Tcm1/1

== system arcelik_a_senem_model/SVPWM/Subsystem5 ==
  Tcm1 : Inport
  Tcm2 : Inport  Port=2
  Tcm3 : Inport  Port=3
  Add : Sum  Inputs=+-
  Add1 : Sum  Inputs=+-
  Add2 : Sum  Inputs=+-
  Relay : Relay
  Relay1 : Relay
  Relay2 : Relay
  Repeating Sequence1 : simulink/Sources/Repeating Sequence  rep_seq_t=[0 Ts/2 Ts]  rep_seq_y=[0 Ts/4 0]
  PWM1 : Outport
  PWM3 : Outport  Port=2
  PWM2 : Outport  Port=3
  wires:
  Repeating Sequence1/1 -> Add1/1, Add2/1, Add/1
  Add2/1 -> Relay2/1
  Relay2/1 -> PWM2/1
  Add1/1 -> Relay1/1
  Relay1/1 -> PWM3/1
  Tcm3/1 -> Add2/2
  Tcm2/1 -> Add1/2
  Tcm1/1 -> Add/2
  Relay/1 -> PWM1/1
  Add/1 -> Relay/1

== system arcelik_a_senem_model/AutoTune/Electrical Parameter Estimation/Electrical Parameter Estimation ==
  Ld : Inport
  R : Inport  Port=2
  Inputs : Inport  Port=3
  Lq : Inport  Port=4
  Enable : EnablePort
  Add : Sum  Inputs=+-
  Bus Selector : BusSelector  OutputSignals=Vq,iq,we,id
  Constant : Constant  Value=Tss
  Divide : Product  Inputs=*/
  Fcn : Fcn  Expr=u(1)-u(6)*u(2)-u(8)*u(5)-u(3)*u(7)*u(4)
  MATLAB Function1 : MATLAB Function  TreatAsAtomicUnit=on
  Mux : Mux  Inputs=8
  Unit Delay : UnitDelay  InitialCondition=0.001  SampleTime=-1  HasFrameUpgradeWarning=on
  Unit Delay1 : UnitDelay  InitialCondition=1e6  SampleTime=-1  HasFrameUpgradeWarning=on
  Unit Delay2 : UnitDelay  SampleTime=-1  HasFrameUpgradeWarning=on
  Unit Delay3 : UnitDelay  SampleTime=-1  HasFrameUpgradeWarning=on
  Flux_linkage_hat : Outport
  wires:
  Divide/1 -> Mux/5
  Constant/1 -> Divide/2
  Add/1 -> Divide/1
  Unit Delay3/1 -> Add/2
  Unit Delay2/1 -> MATLAB Function1/2(InputMatrix)
  Bus Selector/4 -> Mux/4  "<id>"
  Bus Selector/3 -> Unit Delay2/1, Mux/3  "<we>"
  Bus Selector/2 -> Add/1, Unit Delay3/1, Mux/2  "<iq>"
  Bus Selector/1 -> Mux/1  "<Vq>"
  Mux/1 -> Fcn/1
  Fcn/1 -> MATLAB Function1/1(Output)
  Unit Delay/1 -> MATLAB Function1/3(Estimated_1)
  Unit Delay1/1 -> MATLAB Function1/4(CovarianceMatrix_1)
  MATLAB Function1/2(CovarianceMatrix) -> Unit Delay1/1
  MATLAB Function1/1(Estimated) -> Unit Delay/1, Flux_linkage_hat/1
  Inputs/1 -> Bus Selector/1
  R/1 -> Mux/6
  Ld/1 -> Mux/7
  Lq/1 -> Mux/8

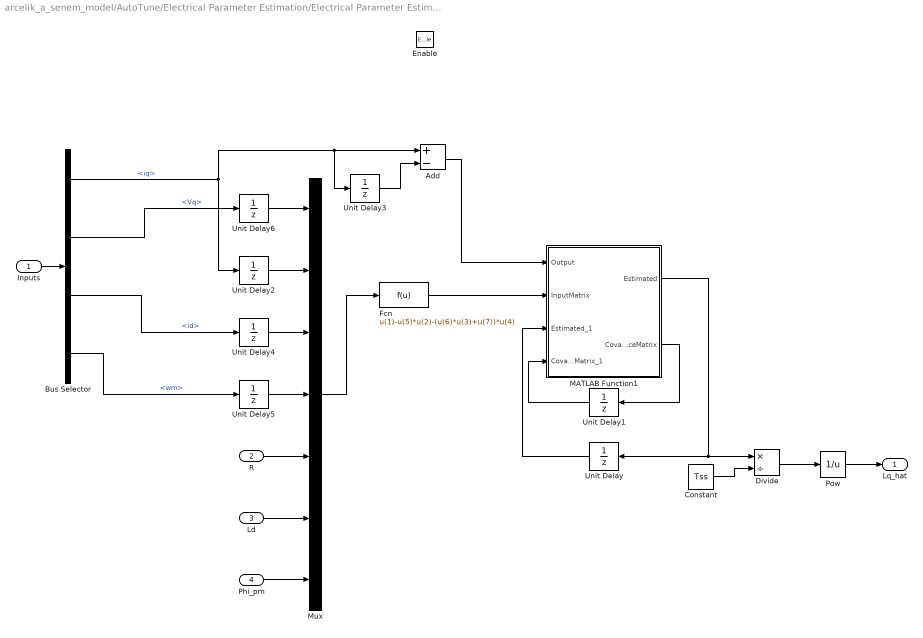
== system arcelik_a_senem_model/AutoTune/Electrical Parameter Estimation/Electrical Parameter Estimation1 ==
  Inputs : Inport
  R : Inport  Port=2
  Ld : Inport  Port=3
  Phi_pm : Inport  Port=4
  Enable : EnablePort
  Add : Sum  Inputs=+-
  Bus Selector : BusSelector  OutputSignals=iq,Vq,id,wm
  Constant : Constant  Value=Tss
  Divide : Product  Inputs=*/
  Fcn : Fcn  Expr=u(1)-u(5)*u(2)-(u(6)*u(3)+u(7))*u(4)
  MATLAB Function1 : MATLAB Function  TreatAsAtomicUnit=on
  Mux : Mux  Inputs=7
  Pow : Math  Operator=reciprocal  RndMeth=Zero  SaturateOnIntegerOverflow=on
  Unit Delay : UnitDelay  InitialCondition=0.01  SampleTime=-1  HasFrameUpgradeWarning=on
  Unit Delay1 : UnitDelay  InitialCondition=1e6  SampleTime=-1  HasFrameUpgradeWarning=on
  Unit Delay{2..6} (5 alike) : UnitDelay  SampleTime=-1  HasFrameUpgradeWarning=on
  Lq_hat : Outport
  wires:
  Unit Delay6/1 -> Mux/1
  Pow/1 -> Lq_hat/1
  Constant/1 -> Divide/2
  Divide/1 -> Pow/1
  Unit Delay5/1 -> Mux/4
  Unit Delay4/1 -> Mux/3
  Unit Delay2/1 -> Mux/2
  Mux/1 -> Fcn/1
  Bus Selector/4 -> Unit Delay5/1  "<wm>"
  Bus Selector/3 -> Unit Delay4/1  "<id>"
  Bus Selector/2 -> Unit Delay6/1  "<Vq>"
  Fcn/1 -> MATLAB Function1/2(InputMatrix)
  Unit Delay3/1 -> Add/2
  Bus Selector/1 -> Add/1, Unit Delay3/1, Unit Delay2/1  "<iq>"
  Add/1 -> MATLAB Function1/1(Output)
  Unit Delay/1 -> MATLAB Function1/3(Estimated_1)
  Unit Delay1/1 -> MATLAB Function1/4(CovarianceMatrix_1)
  MATLAB Function1/2(CovarianceMatrix) -> Unit Delay1/1
  MATLAB Function1/1(Estimated) -> Unit Delay/1, Divide/1
  Inputs/1 -> Bus Selector/1
  R/1 -> Mux/5
  Ld/1 -> Mux/6
  Phi_pm/1 -> Mux/7

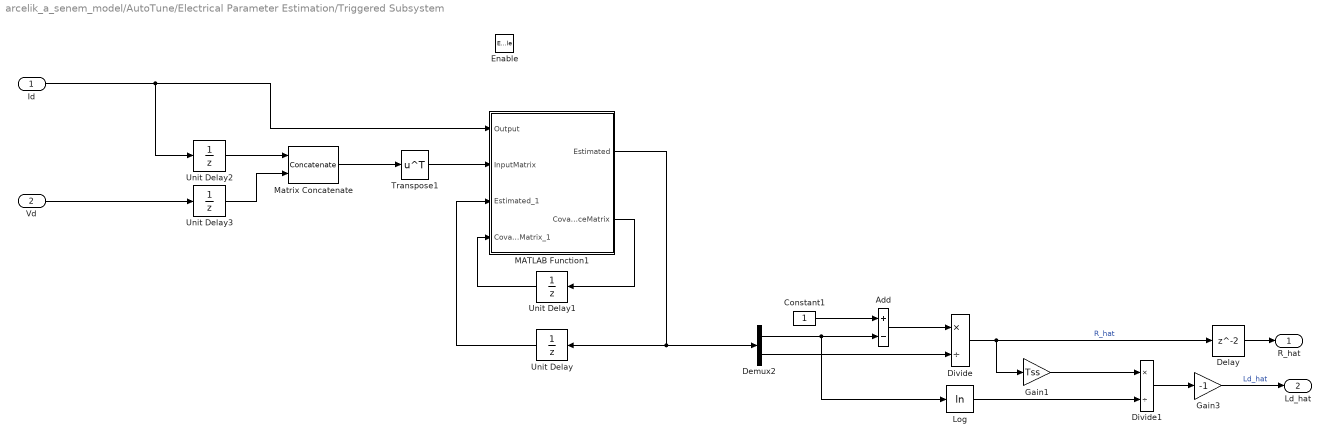
== system arcelik_a_senem_model/AutoTune/Electrical Parameter Estimation/Triggered Subsystem ==
  Id : Inport
  Vd : Inport  Port=2
  Enable : EnablePort
  Add : Sum  Inputs=+-
  Constant1 : Constant
  Delay : Delay
  Demux2 : Demux  Outputs=2
  Divide : Product  Inputs=*/
  Divide1 : Product  Inputs=*/
  Gain1 : Gain  Gain=Tss
  Gain3 : Gain  Gain=-1
  Log : Math  Operator=log  SaturateOnIntegerOverflow=on
  MATLAB Function1 : MATLAB Function
  Matrix Concatenate : Concatenate  Mode=Multidimensional array  ConcatenateDimension=2
  Transpose1 : Math  Operator=transpose  SaturateOnIntegerOverflow=on
  Unit Delay : UnitDelay  InitialCondition=[0.01 ; 0.01]  SampleTime=-1  HasFrameUpgradeWarning=on
  Unit Delay1 : UnitDelay  InitialCondition=[1e6 0; 0 1e6]  SampleTime=-1  HasFrameUpgradeWarning=on
  Unit Delay2 : UnitDelay  SampleTime=-1  HasFrameUpgradeWarning=on
  Unit Delay3 : UnitDelay  SampleTime=-1  HasFrameUpgradeWarning=on
  R_hat : Outport
  Ld_hat : Outport  Port=2
  wires:
  Unit Delay1/1 -> MATLAB Function1/4(CovarianceMatrix_1)
  Demux2/1 -> Add/2, Log/1
  Id/1 -> Unit Delay2/1, MATLAB Function1/1(Output)
  Vd/1 -> Unit Delay3/1
  Constant1/1 -> Add/1
  MATLAB Function1/2(CovarianceMatrix) -> Unit Delay1/1
  Unit Delay2/1 -> Matrix Concatenate/1
  Unit Delay/1 -> MATLAB Function1/3(Estimated_1)
  Divide/1 -> Gain1/1, Delay/1  "R_hat"
  MATLAB Function1/1(Estimated) -> Unit Delay/1, Demux2/1
  Transpose1/1 -> MATLAB Function1/2(InputMatrix)
  Matrix Concatenate/1 -> Transpose1/1
  Add/1 -> Divide/1
  Unit Delay3/1 -> Matrix Concatenate/2
  Gain1/1 -> Divide1/1
  Divide1/1 -> Gain3/1
  Demux2/2 -> Divide/2
  Log/1 -> Divide1/2
  Gain3/1 -> Ld_hat/1  "Ld_hat"
  Delay/1 -> R_hat/1

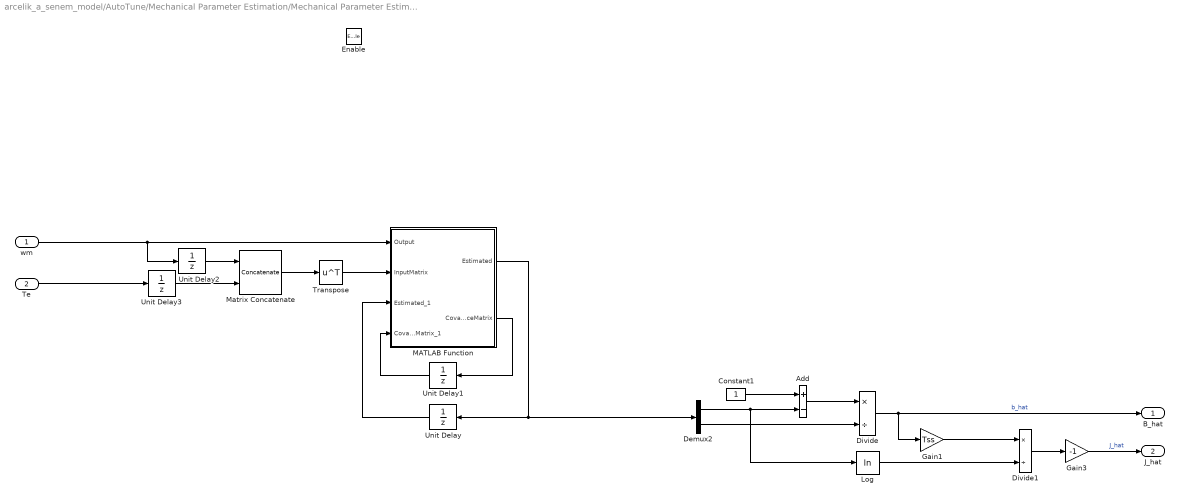
== system arcelik_a_senem_model/AutoTune/Mechanical Parameter Estimation/Mechanical Parameter Estimation ==
  wm : Inport
  Te : Inport  Port=2
  Enable : EnablePort
  Add : Sum  Inputs=+-
  Constant1 : Constant
  Demux2 : Demux  Outputs=2
  Divide : Product  Inputs=*/
  Divide1 : Product  Inputs=*/
  Gain1 : Gain  Gain=Tss
  Gain3 : Gain  Gain=-1
  Log : Math  Operator=log  SaturateOnIntegerOverflow=on
  MATLAB Function : MATLAB Function
  Matrix Concatenate : Concatenate  Mode=Multidimensional array  ConcatenateDimension=2
  Transpose : Math  Operator=transpose  SaturateOnIntegerOverflow=on
  Unit Delay : UnitDelay  InitialCondition=[0.01 ; 0.01]  SampleTime=-1  HasFrameUpgradeWarning=on
  Unit Delay1 : UnitDelay  InitialCondition=[1e6 0; 0 1e6]  SampleTime=-1  HasFrameUpgradeWarning=on
  Unit Delay2 : UnitDelay  SampleTime=-1  HasFrameUpgradeWarning=on
  Unit Delay3 : UnitDelay  SampleTime=-1  HasFrameUpgradeWarning=on
  B_hat : Outport
  J_hat : Outport  Port=2
  wires:
  Unit Delay/1 -> MATLAB Function/3(Estimated_1)
  Divide/1 -> B_hat/1, Gain1/1  "b_hat"
  MATLAB Function/2(CovarianceMatrix) -> Unit Delay1/1
  Constant1/1 -> Add/1
  Unit Delay1/1 -> MATLAB Function/4(CovarianceMatrix_1)
  MATLAB Function/1(Estimated) -> Demux2/1, Unit Delay/1
  Demux2/2 -> Divide/2
  Divide1/1 -> Gain3/1
  Demux2/1 -> Log/1, Add/2
  Gain1/1 -> Divide1/1
  Log/1 -> Divide1/2
  Gain3/1 -> J_hat/1  "J_hat"
  Add/1 -> Divide/1
  Unit Delay2/1 -> Matrix Concatenate/1
  Unit Delay3/1 -> Matrix Concatenate/2
  Matrix Concatenate/1 -> Transpose/1
  Transpose/1 -> MATLAB Function/2(InputMatrix)
  wm/1 -> Unit Delay2/1, MATLAB Function/1(Output)
  Te/1 -> Unit Delay3/1

== system arcelik_a_senem_model/PMSM/Id, Iq Calculation/Id cal ==
  Iq : Inport
  we : Inport  Port=2
  Vd : Inport  Port=3
  1/Ld : Gain  Gain=1/Ld
  Integrator : Integrator
  Lq/Ld : Gain  Gain=Lq
  Product : Product  RndMeth=Zero
  Rs/Ld : Gain  Gain=Rs
  Sum : Sum  Inputs=-++
  Id : Outport
  wires:
  Iq/1 -> Product/1
  we/1 -> Product/2
  Product/1 -> Lq/Ld/1
  Integrator/1 -> Id/1, Rs/Ld/1
  Sum/1 -> 1/Ld/1
  Vd/1 -> Sum/3
  Lq/Ld/1 -> Sum/2
  Rs/Ld/1 -> Sum/1
  1/Ld/1 -> Integrator/1

== system arcelik_a_senem_model/PMSM/Id, Iq Calculation/Iq cal ==
  Id : Inport
  Vq : Inport  Port=2
  we : Inport  Port=3
  1/Lq : Gain  Gain=1/Lq
  Integrator : Integrator
  Ld/Lq : Gain  Gain=Ld
  Product : Product  RndMeth=Zero
  Rs/Lq : Gain  Gain=Rs
  Sum : Sum  Inputs=---+
  shi_f/Lq : Gain  Gain=flux
  Iq : Outport
  wires:
  Rs/Lq/1 -> Sum/1
  Ld/Lq/1 -> Sum/2
  shi_f/Lq/1 -> Sum/3
  Vq/1 -> Sum/4
  Sum/1 -> 1/Lq/1
  Integrator/1 -> Rs/Lq/1, Iq/1
  Product/1 -> Ld/Lq/1
  we/1 -> Product/2, shi_f/Lq/1
  Id/1 -> Product/1
  1/Lq/1 -> Integrator/1

== matlab function arcelik_a_senem_model/AutoTune/Electrical Parameter Estimation/Triggered Subsystem/MATLAB Function1 ==
  data: Estimated output; Output input; CovarianceMatrix output; InputMatrix input; Estimated_1 input; CovarianceMatrix_1 input
function [Estimated,CovarianceMatrix] = RLS(Output,InputMatrix,Estimated_1,CovarianceMatrix_1)

ForgettingFactor = 0.999;
y = Output;
phi = InputMatrix;
e = y - (phi')*Estimated_1;
L = CovarianceMatrix_1*phi/(ForgettingFactor*eye(size(Output)) + (phi')*CovarianceMatrix_1*phi);
CovarianceMatrix = (CovarianceMatrix_1-L*(phi')*CovarianceMatrix_1)/ForgettingFactor;
Estimated = Estimated_1 + L*e;

== matlab function arcelik_a_senem_model/AutoTune/Electrical Parameter Estimation/Electrical Parameter Estimation1/MATLAB Function1 ==
  data: Estimated output; Output input; CovarianceMatrix output; InputMatrix input; Estimated_1 input; CovarianceMatrix_1 input
function [Estimated,CovarianceMatrix] = RLS(Output,InputMatrix,Estimated_1,CovarianceMatrix_1)

ForgettingFactor = 0.999;
y = Output;
phi = InputMatrix;
e = y - (phi')*Estimated_1;
L = CovarianceMatrix_1*phi/(ForgettingFactor*eye(1,1) + (phi')*CovarianceMatrix_1*phi);
CovarianceMatrix = (CovarianceMatrix_1-L*(phi')*CovarianceMatrix_1)/ForgettingFactor;
Estimated = Estimated_1 + L*e;

== matlab function arcelik_a_senem_model/AutoTune/Electrical Parameter Estimation/Electrical Parameter Estimation/MATLAB Function1 ==
  data: Estimated output; Output input; CovarianceMatrix output; InputMatrix input; Estimated_1 input; CovarianceMatrix_1 input
function [Estimated,CovarianceMatrix] = RLS(Output,InputMatrix,Estimated_1,CovarianceMatrix_1)

ForgettingFactor = 0.999;
y = Output;
phi = InputMatrix;
e = y - (phi')*Estimated_1;
L = CovarianceMatrix_1*phi/(ForgettingFactor*eye(1,1) + (phi')*CovarianceMatrix_1*phi);
CovarianceMatrix = (CovarianceMatrix_1-L*(phi')*CovarianceMatrix_1)/ForgettingFactor;
Estimated = Estimated_1 + L*e;

== stateflow chart arcelik_a_senem_model/Chart ==
  state AutotuneOff
    en: tuneoff = 0;
    EstimateStep1 = 0;
    EstimateStep2 = 0;
    EstimateStep3 =0;
    EstimateStep4 = 0;
    Mode=4;
  state AutotuneOn
    state Step1 % Estimate R and Ld
      en: Mode = 1;
      du: EstimateStep1 = 1;
      EstimateStep2 = 0;
      EstimateStep3 = 0;
      EstimateStep4 = 0;
    state Step2 % Estimate Flux Linkage
      en: Mode = 2;
      du: EstimateStep2 =1;
      EstimateStep1 = 0;
      EstimateStep3 = 0;
      EstimateStep4 = 0;
    state MechanicalEstimation
      en: Mode = 3;
      du: EstimateStep4 = 1;
      EstimateStep2 = 0;
      EstimateStep3 = 0;
      EstimateStep1= 0;
    state Step3 % Estimate Lq
      en: Mode  = 2;
      du: EstimateStep3 = 1;
      EstimateStep1 = 0;
      EstimateStep2 =0;
      EstimateStep4 = 0;
    (default) -> Step1 % Estimate R and Ld
    Step1 % Estimate R and Ld -> Step2 % Estimate Flux Linkage : after(1,sec)
    Step2 % Estimate Flux Linkage -> Step3 % Estimate Lq : after(1,sec)
    Step3 % Estimate Lq -> MechanicalEstimation : after(1,sec)
  (default) -> AutotuneOff : {Mode=4;}
  AutotuneOff -> AutotuneOn : [switch_on]
  AutotuneOn -> AutotuneOff : after(5,sec){UpdateGains=1;}
  data: switch_on input; Mode output; EstimateStep1 output; EstimateStep2 output; EstimateStep3 output; tuneoff local; EstimateStep4 output; UpdateGains output

== matlab function arcelik_a_senem_model/AutoTune/Mechanical Parameter Estimation/Mechanical Parameter Estimation/MATLAB Function ==
  data: Estimated output; Output input; CovarianceMatrix output; InputMatrix input; Estimated_1 input; CovarianceMatrix_1 input
function [Estimated,CovarianceMatrix] = RLS(Output,InputMatrix,Estimated_1,CovarianceMatrix_1)

ForgettingFactor = 0.999;
y = Output;
phi = InputMatrix;
e = y - (phi')*Estimated_1;
L = CovarianceMatrix_1*phi/(ForgettingFactor*eye(size(Output)) + (phi')*CovarianceMatrix_1*phi);
CovarianceMatrix = (CovarianceMatrix_1-L*(phi')*CovarianceMatrix_1)/ForgettingFactor;
Estimated = Estimated_1 + L*e;

== matlab function arcelik_a_senem_model/SpeedRef/RC_MACRO1 ==
  settings: updateMethod=DISCRETE  sampleTime=Ts
  data: inp input; SetpointValue output; MaxSpeed input
function SetpointValue = rmp_cntl(inp,MaxSpeed)
%#codegen
TargetValue = inp;         
persistent EqualFlag;       
persistent RampDelayCount;  
persistent SetpointValue_x; 	

RampDelayMax=1e-5;     		
RampLowLimit=-MaxSpeed;    					  
RampHighLimit=MaxSpeed;    	

if isempty(RampDelayCount)
    RampDelayCount=0;    	
end
if isempty(SetpointValue_x)
    SetpointValue_x=0;
end
if isempty(EqualFlag)
    EqualFlag=0;       
end

	rc_tmp = TargetValue - SetpointValue_x;	
%  /*  0.0000305 is resolution of Q15 */ 					
 if (abs(rc_tmp) > 0.00001)	%0.0000305	0.00001 															
	RampDelayCount = RampDelayCount + 1;	
    if (RampDelayCount >= RampDelayMax)															
        if (TargetValue >= SetpointValue_x)												
            SetpointValue_x = SetpointValue_x + 0.001;
        else																				
            SetpointValue_x = SetpointValue_x - 0.001;	
        end
        if (SetpointValue_x > RampHighLimit)
            SetpointValue_x = RampHighLimit;
        elseif (SetpointValue_x < RampLowLimit)		
            SetpointValue_x = RampLowLimit;																									
        end	
        RampDelayCount = 0;
    end
 else
     EqualFlag = 1;
 end   
 SetpointValue = SetpointValue_x;
end


%               _iq    TargetValue; 	// Input: Target input (pu)
%				 Uint32 RampDelayMax;	// Parameter: Maximum delay rate (Q0) - independently with global Q			
%		 	 	 _iq    RampLowLimit;	// Parameter: Minimum limit (pu)				  
%				 _iq    RampHighLimit;	// Parameter: Maximum limit (pu)
%				 Uint32 RampDelayCount; // Variable: Incremental delay (Q0) - independently with global Q	
%				 _iq    SetpointValue;	// Output: Target output (pu)				 
%				 Uint32 EqualFlag;		// Output: Flag output (Q0) - independently with global Q
%				 _iq	rc_tmp;			// Variable: Temp variable

== matlab function arcelik_a_senem_model/InverseParkTransformation/ipark ==
  settings: updateMethod=DISCRETE  sampleTime=Ts
  data: Ds input; Alpha output; Qs input; Angle input; Beta output
function [Alpha,Beta] = ipark(Ds,Qs,Angle)
%#codegen

cosangle = cos(Angle);             
sinangle = sin(Angle);

Alpha = (Ds*cosangle - Qs*sinangle);       
Beta = (Qs*cosangle + Ds*sinangle);         	

end

%                 _iq  Alpha;  		// Output: stationary d-axis stator variable
%				  _iq  Beta;		// Output: stationary q-axis stator variable
%				  _iq  Angle;		// Input: rotating angle (pu)
%				  _iq  Ds;			// Input: rotating d-axis stator variable
%				  _iq  Qs;			// Input: rotating q-axis stator variable
%				  _iq  Sine;		// Input: Sine term
%				  _iq  Cosine;		// Input: Cosine term
